simulink library "library_schuettgut"  (R2020a)
settings: Solver=VariableStepAuto  StartTime=0.0  StopTime=10.0  RelTol=1e-3
undefined symbols (not defined in the file or in its folder): alpha, beta, n_n, T, tau_LV, tau_OL, tau_SK, tau_V
libraries: simulink x9, powerlib_meascontrol x2
settings Model: Creator=Jonathan  LastModifiedBy=Jonathan

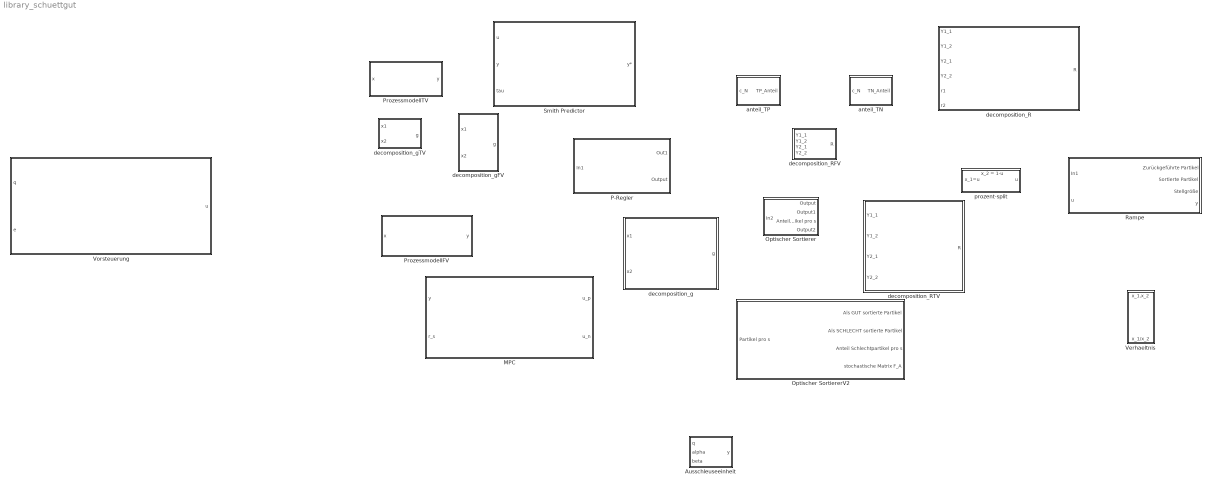
== system library_schuettgut ==
  Ausschleuseeinheit : MATLAB Function  TreatAsAtomicUnit=on
  MPC : Subsystem
  Optischer Sortierer : Subsystem  mask{alpha=0, beta=0}
      mask prompts: alpha "Wahrscheinlichkeit alpha:"; beta "Wahrscheinlichkeit beta:"
  Optischer SortiererV2 : Subsystem  AncestorBlock=library_schuettgut/Optischer Sortierer
  P-Regler : Subsystem  mask{gain=1, delay=1, TrueorFalse=0}
      mask prompts: delay "Time Delay"; TrueorFalse "Reglerinput"
  ProzessmodellFV : Subsystem
  ProzessmodellTV : Subsystem
  Rampe : Subsystem  Tag=Rampe  mask{OK=tau_OL, errorP=0, errorN=0, KV=tau_LV, V=tau_V, TrueorFalse=0, delay=0.2, gain=8.6, KP=6/10000, KN=6/10000}
      mask prompts: OK "Abstand OS Kamera"; errorP "Reglerfehler Gutpartikel:"; errorN "Reglerfehler Schlechtpartikel"; KV "Abstand Kamera Vakuumsauger"; V "Totzeit durch Absaugen"; TrueorFalse "Reglerinput:"; delay "Regler-Totzeit"; gain "Regler-Gain:"; KP "Amplitude des Kameramessrauschen für die positiven Partikel"; KN "Amplitude des Kameramessrauschen für die negativen Partikel"
      mask help:
      | Reglerinput:
      | Reglerinput = 1 => Gutpartikel pro s wird als Regelgröße verwendet
      | Reglerinput = 0 => Schlechtpartike pro s wird als Regelgröße verwendet
      mask TypeOptions TrueorFalse: 0 | 1
      mask DialogControl Regler Prompt: Regler
      mask DialogControl Kamera Prompt: Kamera
  Smith Predictor : Subsystem
  "Verhaeltnis " : Subsystem
  Vorsteuerung : Subsystem
  anteil_TN : MATLAB Function  TreatAsAtomicUnit=on
  anteil_TP : MATLAB Function  TreatAsAtomicUnit=on
  decomposition_R : MATLAB Function  TreatAsAtomicUnit=on
  decomposition_RFV : MATLAB Function  TreatAsAtomicUnit=on
  decomposition_RTV : MATLAB Function  TreatAsAtomicUnit=on
  decomposition_g : MATLAB Function  TreatAsAtomicUnit=on
  decomposition_gFV : MATLAB Function  TreatAsAtomicUnit=on
  decomposition_gTV : MATLAB Function  TreatAsAtomicUnit=on
  prozent-split : Subsystem
      settings: PortSchema="{\"entries\":[{\"content\":{\"sides\":[{\"content\":{\"connectorIds\":[\"In1\"]},\"type\":\"ConnectorPlacement.EquallySpacedRectSide\",\"uuid\":\"ab8511c8-9f1d-48ad-bf24-85fd477f0bdd\"},{\"content\":{\"connectorIds\":[\"Out1\"],\"side\":\"RIGHT\"},\"type\":\"ConnectorPlacement.EquallySpacedRectSide\",\"uuid\":\"9ac1a19a-8176-444e-9f4d-7beffa0184e3\"},{\"content\":{\"connectorIds\":[\"Out2\"],\"side\":\"TOP\"},\"type\":\"ConnectorPlacement.EquallySpacedRectSide\",\"uuid\":\"376c2400-f821-4649-ab16-706a2da6117b\"}]},\"type\":\"ConnectorPlacement.EquallySpacedConnector\",\"uuid\":\"f6e72b2d-0467-4732-a018-d51f3a5db703\"}],\"packageUris\":[\"http://schema.mathworks.com/mf0/Connector/19700101\"],\"version\":\"1.0\"}"

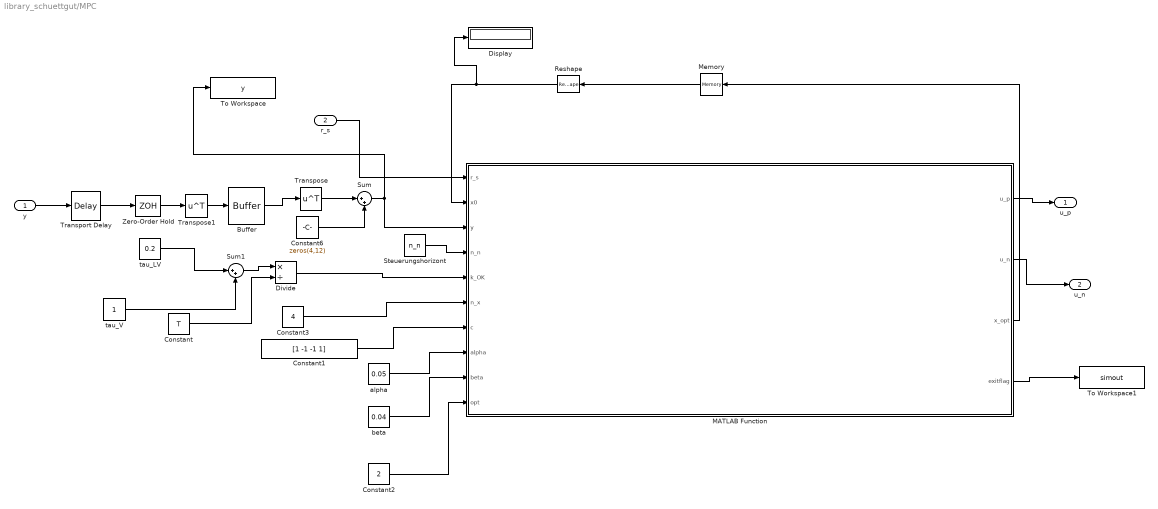
== system library_schuettgut/MPC ==
  y : Inport
  r_s : Inport  Port=2
  Buffer : Buffer  N=n_n  V=n_n-1  OutputFrames=off
  Constant : Constant  Value=T
  Constant1 : Constant  Value=[1 -1 -1 1]
  Constant2 : Constant  Value=2
  Constant3 : Constant  Value=4
  Constant6 : Constant  Value=zeros(4,12)
  Display : Display
  Divide : Product  Inputs=*/
  MATLAB Function : MATLAB Function  TreatAsAtomicUnit=on  SystemSampleTime=T
  Memory : Memory
  Reshape : Reshape  OutputDimensionality=Customize  OutputDimensions=[48,1]
  Steuerungshorizont : Constant  Value=n_n
  Sum : Sum  Inputs=|++
  Sum1 : Sum  Inputs=|++
  To Workspace : ToWorkspace  VariableName=y  SaveFormat=Timeseries  SampleTime=-1
  To Workspace1 : ToWorkspace  VariableName=simout  SaveFormat=Timeseries  SampleTime=-1
  Transport Delay : TransportDelay  DelayTime=tau_SK
  Transpose : Math  Operator=transpose  SaturateOnIntegerOverflow=on
  Transpose1 : Math  Operator=transpose  SaturateOnIntegerOverflow=on
  Zero-Order Hold : ZeroOrderHold  SampleTime=0.1
  alpha : Constant  Value=0.05
  beta : Constant  Value=0.04
  tau_LV : Constant  Value=0.2
  tau_V : Constant
  u_p : Outport
  u_n : Outport  Port=2
  wires:
  r_s/1 -> MATLAB Function/1(r_s)
  MATLAB Function/3(x_opt) -> Memory/1
  alpha/1 -> MATLAB Function/8(alpha)
  beta/1 -> MATLAB Function/9(beta)
  Constant1/1 -> MATLAB Function/7(c)
  Constant3/1 -> MATLAB Function/6(n_x)
  y/1 -> Transport Delay/1
  Zero-Order Hold/1 -> Transpose1/1
  Buffer/1 -> Transpose/1
  Constant6/1 -> Sum/2
  MATLAB Function/2(u_n) -> u_n/1
  MATLAB Function/1(u_p) -> u_p/1
  Transpose1/1 -> Buffer/1
  Memory/1 -> Reshape/1
  Reshape/1 -> MATLAB Function/2(x0), Display/1
  Sum/1 -> To Workspace/1, MATLAB Function/3(y)
  MATLAB Function/4(exitflag) -> To Workspace1/1
  Constant2/1 -> MATLAB Function/10(opt)
  tau_LV/1 -> Sum1/1
  tau_V/1 -> Sum1/2
  Sum1/1 -> Divide/1
  Divide/1 -> MATLAB Function/5(k_OK)
  Constant/1 -> Divide/2
  Transpose/1 -> Sum/1
  Steuerungshorizont/1 -> MATLAB Function/4(n_n)
  Transport Delay/1 -> Zero-Order Hold/1

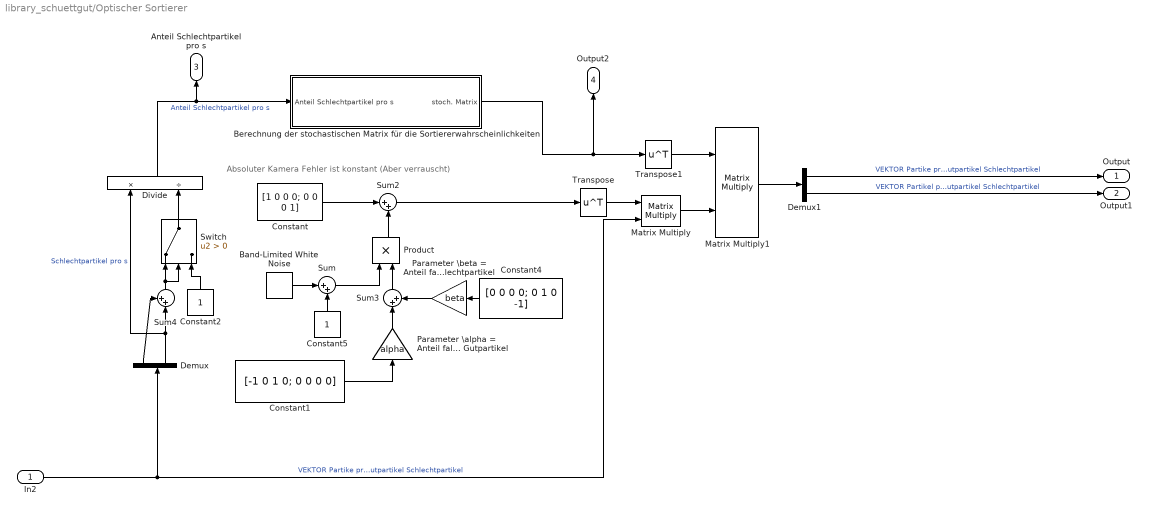
== system library_schuettgut/Optischer Sortierer ==
  note: Absoluter Kamera Fehler ist konstant (Aber verrauscht)
  In2 : Inport
  Band-Limited White Noise : simulink/Sources/Band-Limited White Noise  Cov=[0]  Ts=0.1  seed=[23341]
  Berechnung der stochastischen Matrix für die Sortiererwahrscheinlichkeiten : Subsystem
  Constant : Constant  Value=[1 0 0 0; 0 0 0 1]
  Constant1 : Constant  Value=[-1 0 1 0; 0 0 0 0]
  Constant2 : Constant
  Constant4 : Constant  Value=[0 0 0 0; 0 1 0 -1]
  Constant5 : Constant
  Demux : Demux  Outputs=2
  Demux1 : Demux  Outputs=2
  Divide : Product  Inputs=*/
  Matrix Multiply : Product  Multiplication=Matrix(*)
  Matrix Multiply1 : Product  Multiplication=Matrix(*)
  Parameter \alpha = Anteil falsch detektierter Gutpartikel : Gain  Gain=alpha
  Parameter \beta = Anteil falsch detektierter Schlechtpartikel : Gain  Gain=beta
  Product : Product
  Sum : Sum  Inputs=|++
  Sum2 : Sum  Inputs=|++
  Sum3 : Sum  Inputs=|++
  Sum4 : Sum  Inputs=++|
  Switch : Switch  Criteria=u2 > Threshold
  Transpose : Math  Operator=transpose  SaturateOnIntegerOverflow=on
  Transpose1 : Math  Operator=transpose  SaturateOnIntegerOverflow=on
  Output : Outport
  Output1 : Outport  Port=2
  Anteil Schlechtpartikel pro s : Outport  Port=3
  Output2 : Outport  Port=4
  wires:
  Constant2/1 -> Switch/3
  Switch/1 -> Divide/2
  Constant5/1 -> Sum/2
  Band-Limited White Noise/1 -> Sum/1
  Sum/1 -> Product/1
  Product/1 -> Sum2/2
  Constant/1 -> Sum2/1
  Sum3/1 -> Product/2
  Parameter \alpha = Anteil falsch detektierter Gutpartikel/1 -> Sum3/1
  Parameter \beta = Anteil falsch detektierter Schlechtpartikel/1 -> Sum3/2
  Constant4/1 -> Parameter \beta = Anteil falsch detektierter Schlechtpartikel/1
  Berechnung der stochastischen Matrix für die Sortiererwahrscheinlichkeiten/1(stoch. Matrix) -> Transpose1/1, Output2/1
  Divide/1 -> Berechnung der stochastischen Matrix für die Sortiererwahrscheinlichkeiten/1(Anteil Schlechtpartikel pro s), Anteil Schlechtpartikel pro s/1  "Anteil Schlechtpartikel pro s"
  Demux/1 -> Sum4/1
  Sum4/1 -> Switch/1, Switch/2
  Demux/2 -> Sum4/2, Divide/1  "Schlechtpartikel pro s"
  Sum2/1 -> Transpose/1
  Constant1/1 -> Parameter \alpha = Anteil falsch detektierter Gutpartikel/1
  In2/1 -> Demux/1, Matrix Multiply/2  "VEKTOR Partike pro s: Gutpartikel Schlechtpartikel"
  Matrix Multiply1/1 -> Demux1/1
  Transpose1/1 -> Matrix Multiply1/1
  Matrix Multiply/1 -> Matrix Multiply1/2
  Transpose/1 -> Matrix Multiply/1
  Demux1/2 -> Output1/1  "VEKTOR Partikel pro s in der Schlechtfraktion: Gutpartikel Schlechtpartikel"
  Demux1/1 -> Output/1  "VEKTOR Partike pro s in der Gutfraktion: Gutpartikel Schlechtpartikel"

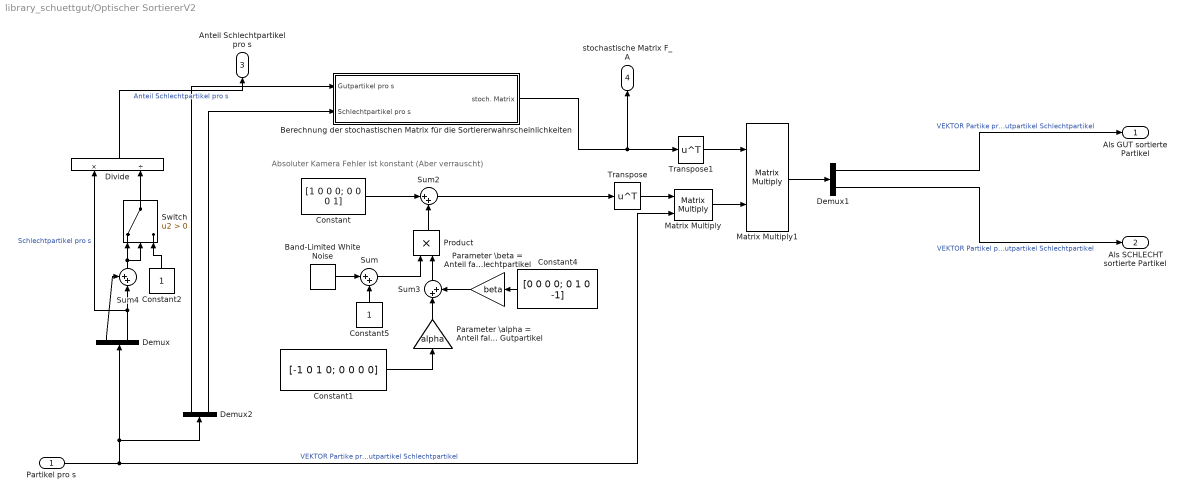
== system library_schuettgut/Optischer SortiererV2 ==
  note: Absoluter Kamera Fehler ist konstant (Aber verrauscht)
  Partikel pro s : Inport
  Band-Limited White Noise : simulink/Sources/Band-Limited White Noise  Cov=[0]  Ts=0.1  seed=[23341]
  Berechnung der stochastischen Matrix für die Sortiererwahrscheinlichkeiten : Subsystem
  Constant : Constant  Value=[1 0 0 0; 0 0 0 1]
  Constant1 : Constant  Value=[-1 0 1 0; 0 0 0 0]
  Constant2 : Constant
  Constant4 : Constant  Value=[0 0 0 0; 0 1 0 -1]
  Constant5 : Constant
  Demux : Demux  Outputs=2
  Demux1 : Demux  Outputs=2
  Demux2 : Demux  Outputs=2
  Divide : Product  Inputs=*/
  Matrix Multiply : Product  Multiplication=Matrix(*)
  Matrix Multiply1 : Product  Multiplication=Matrix(*)
  Parameter \alpha = Anteil falsch detektierter Gutpartikel : Gain  Gain=alpha
  Parameter \beta = Anteil falsch detektierter Schlechtpartikel : Gain  Gain=beta
  Product : Product
  Sum : Sum  Inputs=|++
  Sum2 : Sum  Inputs=|++
  Sum3 : Sum  Inputs=|++
  Sum4 : Sum  Inputs=++|
  Switch : Switch  Criteria=u2 > Threshold
  Transpose : Math  Operator=transpose  SaturateOnIntegerOverflow=on
  Transpose1 : Math  Operator=transpose  SaturateOnIntegerOverflow=on
  Als GUT sortierte Partikel : Outport
  Als SCHLECHT sortierte Partikel : Outport  Port=2
  Anteil Schlechtpartikel pro s : Outport  Port=3
  stochastische Matrix F_A : Outport  Port=4
  wires:
  Demux1/1 -> Als GUT sortierte Partikel/1  "VEKTOR Partike pro s in der Gutfraktion: Gutpartikel Schlechtpartikel"
  Demux1/2 -> Als SCHLECHT sortierte Partikel/1  "VEKTOR Partikel pro s in der Schlechtfraktion: Gutpartikel Schlechtpartikel"
  Transpose/1 -> Matrix Multiply/1
  Matrix Multiply/1 -> Matrix Multiply1/2
  Transpose1/1 -> Matrix Multiply1/1
  Matrix Multiply1/1 -> Demux1/1
  Partikel pro s/1 -> Matrix Multiply/2, Demux2/1, Demux/1  "VEKTOR Partike pro s: Gutpartikel Schlechtpartikel"
  Constant1/1 -> Parameter \alpha = Anteil falsch detektierter Gutpartikel/1
  Sum2/1 -> Transpose/1
  Demux/2 -> Divide/1, Sum4/2  "Schlechtpartikel pro s"
  Sum4/1 -> Switch/2, Switch/1
  Demux/1 -> Sum4/1
  Divide/1 -> Anteil Schlechtpartikel pro s/1  "Anteil Schlechtpartikel pro s"
  Berechnung der stochastischen Matrix für die Sortiererwahrscheinlichkeiten/1(stoch. Matrix) -> stochastische Matrix F_A/1, Transpose1/1
  Constant4/1 -> Parameter \beta = Anteil falsch detektierter Schlechtpartikel/1
  Parameter \beta = Anteil falsch detektierter Schlechtpartikel/1 -> Sum3/2
  Parameter \alpha = Anteil falsch detektierter Gutpartikel/1 -> Sum3/1
  Sum3/1 -> Product/2
  Constant/1 -> Sum2/1
  Product/1 -> Sum2/2
  Sum/1 -> Product/1
  Band-Limited White Noise/1 -> Sum/1
  Constant5/1 -> Sum/2
  Switch/1 -> Divide/2
  Constant2/1 -> Switch/3
  Demux2/1 -> Berechnung der stochastischen Matrix für die Sortiererwahrscheinlichkeiten/1(Gutpartikel pro s)
  Demux2/2 -> Berechnung der stochastischen Matrix für die Sortiererwahrscheinlichkeiten/2(Schlechtpartikel pro s)

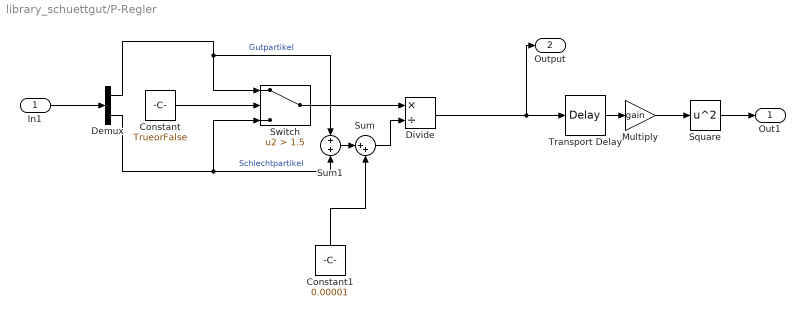
== system library_schuettgut/P-Regler ==
  In1 : Inport
  Constant : Constant  Value=TrueorFalse
  Constant1 : Constant  Value=0.00001
  Demux : Demux  Outputs=2
  Divide : Product  Inputs=*/
  Multiply : Gain  Gain=gain
  Square : Math  Operator=square  SaturateOnIntegerOverflow=on
  Sum : Sum  Inputs=|++
  Sum1 : Sum  Inputs=+|+
  Switch : Switch  Criteria=u2 > Threshold  Threshold=1.5
  Transport Delay : TransportDelay  DelayTime=delay
  Out1 : Outport
  Output : Outport  Port=2
  wires:
  In1/1 -> Demux/1
  Demux/2 -> Switch/3, Sum1/2  "Schlechtpartikel"
  Transport Delay/1 -> Multiply/1
  Multiply/1 -> Square/1
  Constant/1 -> Switch/2
  Demux/1 -> Sum1/1, Switch/1  "Gutpartikel"
  Sum1/1 -> Sum/1
  Sum/1 -> Divide/2
  Constant1/1 -> Sum/2
  Switch/1 -> Divide/1
  Divide/1 -> Transport Delay/1, Output/1
  Square/1 -> Out1/1

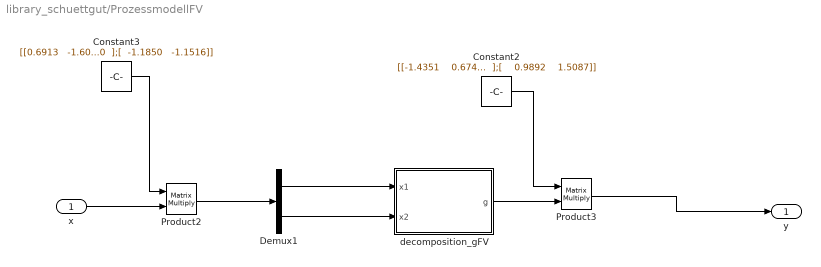
== system library_schuettgut/ProzessmodellFV ==
  x : Inport
  Constant2 : Constant  Value=|
      | [[-1.4351    0.6740
      |  ];[    0.9892    1.5087]]
  Constant3 : Constant  Value=|
      | [[0.6913   -1.6000
      |  ];[  -1.1850   -1.1516]]
  Demux1 : Demux  Outputs=2
  Product2 : Product  Multiplication=Matrix(*)
  Product3 : Product  Multiplication=Matrix(*)
  decomposition_gFV : MATLAB Function  TreatAsAtomicUnit=on
  y : Outport
  wires:
  Constant3/1 -> Product2/1
  Product2/1 -> Demux1/1
  Product3/1 -> y/1
  Constant2/1 -> Product3/1
  Demux1/2 -> decomposition_gFV/2(x2)
  Demux1/1 -> decomposition_gFV/1(x1)
  decomposition_gFV/1(g) -> Product3/2
  x/1 -> Product2/2

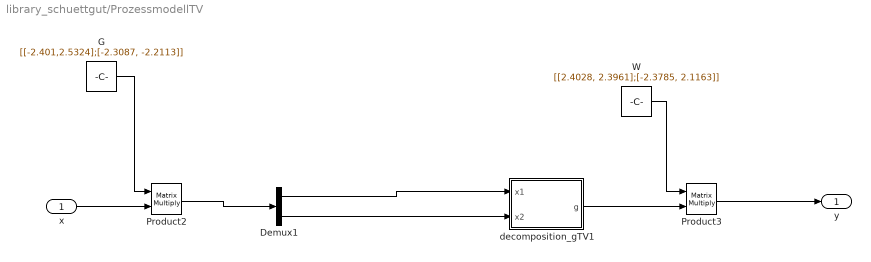
== system library_schuettgut/ProzessmodellTV ==
  x : Inport
  Demux1 : Demux  Outputs=2
  G : Constant  Value=[[-2.401,2.5324];[-2.3087, -2.2113]]
  Product2 : Product  Multiplication=Matrix(*)
  Product3 : Product  Multiplication=Matrix(*)
  W : Constant  Value=[[2.4028, 2.3961];[-2.3785, 2.1163]]
  decomposition_gTV1 : MATLAB Function  TreatAsAtomicUnit=on
  y : Outport
  wires:
  G/1 -> Product2/1
  Demux1/1 -> decomposition_gTV1/1(x1)
  Product3/1 -> y/1
  Product2/1 -> Demux1/1
  x/1 -> Product2/2
  Demux1/2 -> decomposition_gTV1/2(x2)
  W/1 -> Product3/1
  decomposition_gTV1/1(g) -> Product3/2

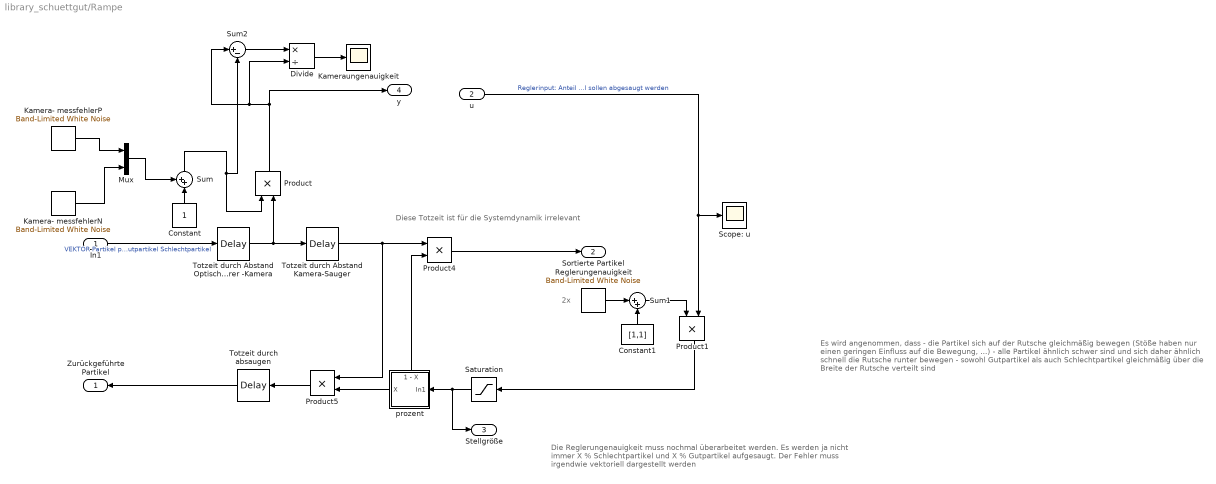
== system library_schuettgut/Rampe ==
  note: Diese Totzeit ist für die Systemdynamik irrelevant
  note: 2x
  note: Die Reglerungenauigkeit muss nochmal überarbeitet werden.
      | Es werden ja nicht immer X % Schlechtpartikel und X %
      | Gutpartikel aufgesaugt. Der Fehler muss irgendwie vektoriell dargestellt werden
  note: Es wird angenommen, dass
      | - die Partikel sich auf der Rutsche gleichmäßig bewegen (Stöße haben nur einen geringen Einfluss auf die Bewegung, ...)
      | - alle Partikel ähnlich schwer sind und sich daher ähnlich schnell die Rutsche runter bewegen
      | - sowohl Gutpartikel als auch Schlechtpartikel gleichmäßig über die Breite der Rutsche verteilt sind
  In1 : Inport
  u : Inport  Port=2
  Constant : Constant
  Constant1 : Constant  Value=[1,1]
  Divide : Product  Inputs=*/
  Kamera- messfehlerN : simulink/Sources/Band-Limited White Noise  Cov=[KN]  Ts=0.6  seed=[242211]
  Kamera- messfehlerP : simulink/Sources/Band-Limited White Noise  Cov=[KP]  Ts=0.6  seed=[15432]
  Kameraungenauigkeit : Scope
  Mux : Mux  Inputs=2
  Product : Product
  Product1 : Product  OutMin=0  OutMax=1
  Product4 : Product
  Product5 : Product
  Reglerungenauigkeit : simulink/Sources/Band-Limited White Noise  Cov=[errorP errorN]  Ts=0.1  seed=[23341]
  Saturation : Saturate  UpperLimit=1  LowerLimit=0
  Scope: u : Scope
  Sum : Sum  Inputs=++|
  Sum1 : Sum  Inputs=|++
  Sum2 : Sum  Inputs=|+-
  Totzeit durch Abstand Optischer Sortierer -Kamera : TransportDelay  DelayTime=OK
  Totzeit durch Abstand Kamera-Sauger : TransportDelay  DelayTime=KV
  Totzeit durch absaugen : TransportDelay  DelayTime=V
  prozent : Subsystem
      settings: PortSchema="{\"entries\":[{\"content\":{\"sides\":[{\"content\":{\"connectorIds\":[\"In1\"]},\"type\":\"ConnectorPlacement.EquallySpacedRectSide\",\"uuid\":\"ab8511c8-9f1d-48ad-bf24-85fd477f0bdd\"},{\"content\":{\"connectorIds\":[\"Out1\"],\"side\":\"RIGHT\"},\"type\":\"ConnectorPlacement.EquallySpacedRectSide\",\"uuid\":\"9ac1a19a-8176-444e-9f4d-7beffa0184e3\"},{\"content\":{\"connectorIds\":[\"Out2\"],\"side\":\"TOP\"},\"type\":\"ConnectorPlacement.EquallySpacedRectSide\",\"uuid\":\"376c2400-f821-4649-ab16-706a2da6117b\"}]},\"type\":\"ConnectorPlacement.EquallySpacedConnector\",\"uuid\":\"f6e72b2d-0467-4732-a018-d51f3a5db703\"}],\"packageUris\":[\"http://schema.mathworks.com/mf0/Connector/19700101\"],\"version\":\"1.0\"}"
  Zurückgeführte Partikel : Outport
  Sortierte Partikel : Outport  Port=2
  Stellgröße : Outport  Port=3
  y : Outport  Port=4
  wires:
  prozent/2(1 - X) -> Product4/2
  prozent/1(X) -> Product5/2
  In1/1 -> Totzeit durch Abstand Optischer Sortierer -Kamera/1  "VEKTOR Partikel pro s: Gutpartikel Schlechtpartikel"
  Product/1 -> Divide/2, Sum2/1, y/1
  Totzeit durch absaugen/1 -> Zurückgeführte Partikel/1
  Totzeit durch Abstand Optischer Sortierer -Kamera/1 -> Totzeit durch Abstand Kamera-Sauger/1, Product/2
  Product5/1 -> Totzeit durch absaugen/1
  Product4/1 -> Sortierte Partikel/1
  Kamera- messfehlerN/1 -> Mux/2
  u/1 -> Scope: u/1, Product1/2  "Reglerinput: Anteil X der Partikel sollen abgesaugt werden"
  Constant/1 -> Sum/2
  Sum/1 -> Sum2/2, Product/1
  Reglerungenauigkeit/1 -> Sum1/1
  Constant1/1 -> Sum1/2
  Product1/1 -> Saturation/1
  Saturation/1 -> Stellgröße/1, prozent/1(In1)
  Sum1/1 -> Product1/1
  Totzeit durch Abstand Kamera-Sauger/1 -> Product4/1, Product5/1
  Kamera- messfehlerP/1 -> Mux/1
  Mux/1 -> Sum/1
  Sum2/1 -> Divide/1
  Divide/1 -> Kameraungenauigkeit/1

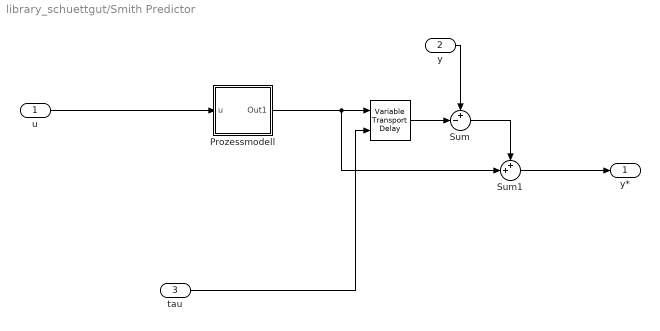
== system library_schuettgut/Smith Predictor ==
  u : Inport
  y : Inport  Port=2
  tau : Inport  Port=3
  " " : VariableTransportDelay  VariableDelayType=Variable transport delay  MaximumDelay=10  MaximumPoints=30000
  Prozessmodell : Subsystem
  Sum : Sum  Inputs=+-|
  Sum1 : Sum  Inputs=++|
  y* : Outport
  wires:
  Prozessmodell/1(Out1) -> Sum1/2, " "/1
  " "/1 -> Sum/2
  y/1 -> Sum/1
  Sum1/1 -> y*/1
  Sum/1 -> Sum1/1
  tau/1 -> " "/2
  u/1 -> Prozessmodell/1(u)

== system library_schuettgut/Verhaeltnis  ==
  x_1,x_2 : Inport
  Demux : Demux  Outputs=2
  Divide : Product  Inputs=*/
  Sum : Sum  Inputs=++|
  x_1/x_2 : Outport
  wires:
  Divide/1 -> x_1/x_2/1
  Demux/2 -> Sum/2
  Demux/1 -> Divide/1, Sum/1
  x_1,x_2/1 -> Demux/1
  Sum/1 -> Divide/2

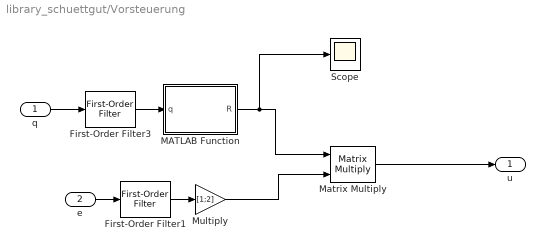
== system library_schuettgut/Vorsteuerung ==
  q : Inport
  e : Inport  Port=2
  First-Order Filter1 : powerlib_meascontrol/Filters/First-Order Filter  FilterType=Lowpass  Tc=200  Ts=0  Initialize=off  Vac_Init=[0, 0, 60]  Vdc_Init=0  PlotResponse=off  FreqRange="[0,  200,  1]"
  First-Order Filter3 : powerlib_meascontrol/Filters/First-Order Filter  FilterType=Lowpass  Tc=200  Ts=0  Initialize=off  Vac_Init=[0, 0, 60]  Vdc_Init=0  PlotResponse=off  FreqRange="[0,  200,  1]"
  MATLAB Function : MATLAB Function  TreatAsAtomicUnit=on
  Matrix Multiply : Product  Multiplication=Matrix(*)
  Multiply : Gain  Gain=[1;2]
  Scope : Scope
  u : Outport
  wires:
  MATLAB Function/1(R) -> Scope/1, Matrix Multiply/1
  q/1 -> First-Order Filter3/1
  Matrix Multiply/1 -> u/1
  e/1 -> First-Order Filter1/1
  Multiply/1 -> Matrix Multiply/2
  First-Order Filter3/1 -> MATLAB Function/1(q)
  First-Order Filter1/1 -> Multiply/1

== system library_schuettgut/prozent-split ==
  u : Inport
  Constant3 : Constant
  Sum7 : Sum  Inputs=|-+
  x_1=u : Outport
  x_2 = 1-u : Outport  Port=2
  wires:
  Constant3/1 -> Sum7/2
  u/1 -> Sum7/1, x_1=u/1  "Reglerinput"
  Sum7/1 -> x_2 = 1-u/1

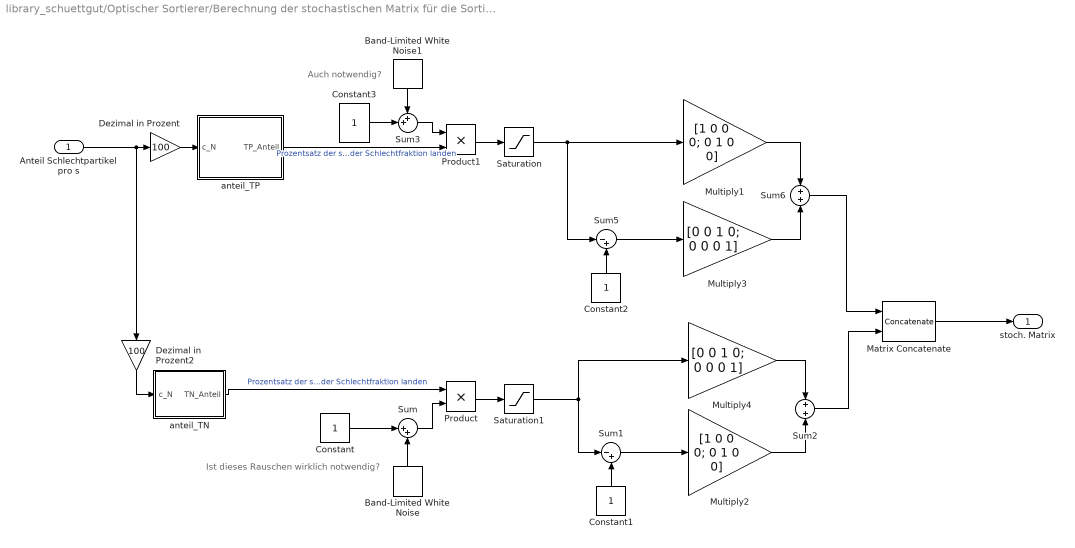
== system library_schuettgut/Optischer Sortierer/Berechnung der stochastischen Matrix für die Sortiererwahrscheinlichkeiten ==
  note: Ist dieses Rauschen wirklich notwendig?
  note: Auch notwendig?
  Anteil Schlechtpartikel pro s : Inport
  Band-Limited White Noise : simulink/Sources/Band-Limited White Noise  Cov=[0]  Ts=0.1  seed=[23341]
  Band-Limited White Noise1 : simulink/Sources/Band-Limited White Noise  Cov=[0]  Ts=0.1  seed=[23341]
  Constant{,1..3} (4 alike) : Constant
  Dezimal in Prozent : Gain  Gain=100
  Dezimal in Prozent2 : Gain  Gain=100
  Matrix Concatenate : Concatenate  Mode=Multidimensional array
  Multiply1 : Gain  Gain=[1 0 0 0; 0 1 0 0]
  Multiply2 : Gain  Gain=[1 0 0 0; 0 1 0 0]
  Multiply3 : Gain  Gain=[0 0 1 0; 0 0 0 1]
  Multiply4 : Gain  Gain=[0 0 1 0; 0 0 0 1]
  Product : Product
  Product1 : Product
  Saturation : Saturate  UpperLimit=1  LowerLimit=0
  Saturation1 : Saturate  UpperLimit=1  LowerLimit=0
  Sum : Sum  Inputs=|++
  Sum1 : Sum  Inputs=|-+
  Sum2 : Sum  Inputs=+|+
  Sum3 : Sum  Inputs=++|
  Sum5 : Sum  Inputs=|-+
  Sum6 : Sum  Inputs=+|+
  anteil_TN : MATLAB Function  TreatAsAtomicUnit=on
  anteil_TP : MATLAB Function  TreatAsAtomicUnit=on
  stoch. Matrix : Outport
  wires:
  Band-Limited White Noise/1 -> Sum/2
  Product/1 -> Saturation1/1
  Product1/1 -> Saturation/1
  Band-Limited White Noise1/1 -> Sum3/1
  anteil_TP/1(TP_Anteil) -> Product1/2  "Prozentsatz der schlecht detektierten Partikel, die in der Schlechtfraktion landen"
  anteil_TN/1(TN_Anteil) -> Product/1  "Prozentsatz der schlecht detektierten Partikel, die in der Schlechtfraktion landen"
  Constant3/1 -> Sum3/2
  Sum3/1 -> Product1/1
  Constant/1 -> Sum/1
  Sum/1 -> Product/2
  Dezimal in Prozent2/1 -> anteil_TN/1(c_N)
  Dezimal in Prozent/1 -> anteil_TP/1(c_N)
  Saturation/1 -> Multiply1/1, Sum5/1
  Saturation1/1 -> Sum1/1, Multiply4/1
  Sum6/1 -> Matrix Concatenate/1
  Sum2/1 -> Matrix Concatenate/2
  Matrix Concatenate/1 -> stoch. Matrix/1
  Multiply1/1 -> Sum6/1
  Anteil Schlechtpartikel pro s/1 -> Dezimal in Prozent2/1, Dezimal in Prozent/1
  Multiply4/1 -> Sum2/1
  Multiply2/1 -> Sum2/2
  Constant1/1 -> Sum1/2
  Sum1/1 -> Multiply2/1
  Constant2/1 -> Sum5/2
  Sum5/1 -> Multiply3/1
  Multiply3/1 -> Sum6/2

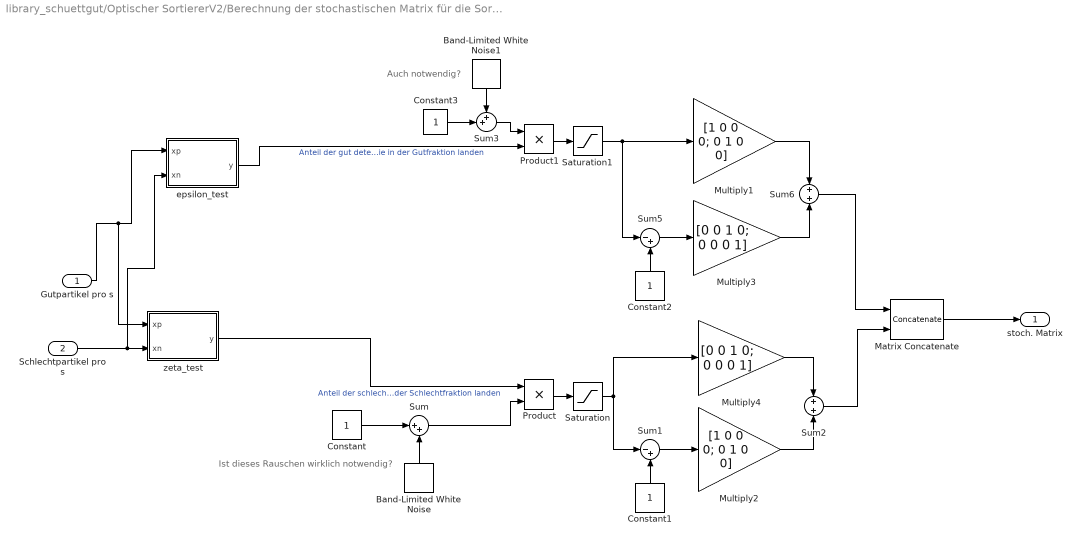
== system library_schuettgut/Optischer SortiererV2/Berechnung der stochastischen Matrix für die Sortiererwahrscheinlichkeiten ==
  note: Auch notwendig?
  note: Ist dieses Rauschen wirklich notwendig?
  Gutpartikel pro s : Inport
  Schlechtpartikel pro s : Inport  Port=2
  Band-Limited White Noise : simulink/Sources/Band-Limited White Noise  Cov=[0]  Ts=0.1  seed=[23341]
  Band-Limited White Noise1 : simulink/Sources/Band-Limited White Noise  Cov=[0]  Ts=0.1  seed=[23341]
  Constant{,1..3} (4 alike) : Constant
  Matrix Concatenate : Concatenate  Mode=Multidimensional array
  Multiply1 : Gain  Gain=[1 0 0 0; 0 1 0 0]
  Multiply2 : Gain  Gain=[1 0 0 0; 0 1 0 0]
  Multiply3 : Gain  Gain=[0 0 1 0; 0 0 0 1]
  Multiply4 : Gain  Gain=[0 0 1 0; 0 0 0 1]
  Product : Product
  Product1 : Product
  Saturation : Saturate  UpperLimit=1  LowerLimit=0
  Saturation1 : Saturate  UpperLimit=1  LowerLimit=0
  Sum : Sum  Inputs=|++
  Sum1 : Sum  Inputs=|-+
  Sum2 : Sum  Inputs=+|+
  Sum3 : Sum  Inputs=++|
  Sum5 : Sum  Inputs=|-+
  Sum6 : Sum  Inputs=+|+
  epsilon_test : MATLAB Function  TreatAsAtomicUnit=on
  zeta_test : MATLAB Function  TreatAsAtomicUnit=on
  stoch. Matrix : Outport
  wires:
  Multiply3/1 -> Sum6/2
  Sum5/1 -> Multiply3/1
  Constant2/1 -> Sum5/2
  Sum1/1 -> Multiply2/1
  Constant1/1 -> Sum1/2
  Multiply2/1 -> Sum2/2
  Multiply4/1 -> Sum2/1
  Multiply1/1 -> Sum6/1
  Matrix Concatenate/1 -> stoch. Matrix/1
  Sum2/1 -> Matrix Concatenate/2
  Sum6/1 -> Matrix Concatenate/1
  Product/1 -> Saturation/1
  Product1/1 -> Saturation1/1
  Sum/1 -> Product/2
  Constant/1 -> Sum/1
  Sum3/1 -> Product1/1
  Constant3/1 -> Sum3/2
  zeta_test/1(y) -> Product/1  "Anteil der schlecht detektierten Partikel, die in der Schlechtfraktion landen"
  epsilon_test/1(y) -> Product1/2  "Anteil der gut detektierten Partikel, die in der Gutfraktion landen"
  Band-Limited White Noise1/1 -> Sum3/1
  Band-Limited White Noise/1 -> Sum/2
  Gutpartikel pro s/1 -> zeta_test/1(xp), epsilon_test/1(xp)
  Schlechtpartikel pro s/1 -> zeta_test/2(xn), epsilon_test/2(xn)
  Saturation/1 -> Multiply4/1, Sum1/1
  Saturation1/1 -> Sum5/1, Multiply1/1

== system library_schuettgut/Rampe/prozent ==
  In1 : Inport
  Constant3 : Constant
  Sum7 : Sum  Inputs=|-+
  X : Outport
  1 - X : Outport  Port=2
  wires:
  Constant3/1 -> Sum7/2
  In1/1 -> Sum7/1, X/1  "Reglerinput"
  Sum7/1 -> 1 - X/1

== system library_schuettgut/Smith Predictor/Prozessmodell ==
  u : Inport
  Out1 : Outport
  wires:
  u/1 -> Out1/1

== matlab function library_schuettgut/decomposition_g ==
  data: x1 input; g output; x2 input
function g = decomposition_g(x1,x2)
%#codegen

%    This function was generated by the Symbolic Math Toolbox version 8.5.
%    23-Jan-2021 16:21:08

t2 = conj(x1);
t3 = conj(x2);
g = [t2.*7.356750433682986e-2-t2.^2.*1.321341967872517e-2+7.302013683153394e-1;t3.*(-6.207010509479585e-2)-t3.^2.*6.60820597936792e-3+8.465045474029088e-1];

== matlab function library_schuettgut/decomposition_R ==
  data: Y1_1 input; R output; Y1_2 input; Y2_1 input; Y2_2 input; r1 input; r2 input
function R = decomposition_R(Y1_1,Y1_2,Y2_1,Y2_2,r1,r2)
%#codegen

%    This function was generated by the Symbolic Math Toolbox version 8.5.
%    23-Jan-2021 16:21:20

t2 = Y1_1.*Y2_2;
t3 = Y1_2.*Y2_1;
t4 = -t3;
t5 = t2+t4;
t6 = 1.0./t5;
R = reshape([r1.*(Y1_1.*t6.*4.209654314594556e-1-Y1_2.*t6.*2.514923794238454e-1-Y2_1.*t6.*2.36103808622674e-1+Y2_2.*t6.*1.41052695029348e-1), ...
r1.*(Y1_1.*t6.*1.329681620461174e-1-Y1_2.*t6.*5.885251943491074e-1-Y2_1.*t6.*7.457688241954584e-2+Y2_2.*t6.*3.300818296991368e-1),...
-r2.*(Y1_1.*t6.*9.471435133466113e-2-Y1_2.*t6.*5.658407033603224e-2-Y2_1.*t6.*5.862694938528591e-1+Y2_2.*t6.*3.502480226974876e-1),...
-r2.*(Y1_1.*t6.*2.991692969348502e-2-Y1_2.*t6.*1.324141553229882e-1-Y2_1.*t6.*1.851818967440092e-1+Y2_2.*t6.*8.196263684039293e-1)],[2,2]);
R(isnan(R))=0;
R(isinf(R))=100;

== matlab function library_schuettgut/decomposition_RTV ==
  data: Y1_1 input; R output; Y1_2 input; Y2_1 input; Y2_2 input
function R = decomposition_RTV(Y1_1,Y1_2,Y2_1,Y2_2)
%#codegen

%    This function was generated by the Symbolic Math Toolbox version 8.5.
%    26-Jan-2021 10:32:41

R = reshape([Y1_2.*(-2.137674923372295e-1)-Y2_2.*2.047522987447861e-1,Y1_1.*2.137674923372295e-1+Y2_1.*2.047522987447861e-1,Y1_2.*2.074157501900618e-1-Y2_2.*2.344807267266782e-1,Y1_1.*(-2.074157501900618e-1)+Y2_1.*2.344807267266782e-1],[2,2]);

== matlab function library_schuettgut/Vorsteuerung/MATLAB Function ==
  data: q input; R output
function R = fcn(q)
% q ist ein 4x1 Vektor mit q_TP,q_FP,q_FN,q_TN
Q_det = 1/(q(1)*q(4)-q(2)*q(3));
R = Q_det*[[q(4) -q(3)];[-q(2) q(1)]];
R(isnan(R)) = 0;
R(isinf(R)) = 10;

== matlab function library_schuettgut/decomposition_RFV ==
  data: Y1_1 input; R output; Y1_2 input; Y2_1 input; Y2_2 input
function R = decomposition_RFV(Y1_1,Y1_2,Y2_1,Y2_2)
%#codegen

%    This function was generated by the Symbolic Math Toolbox version 8.5.
%    27-Jan-2021 00:16:44

t2 = Y1_1.*Y2_2;
t3 = Y1_2.*Y2_1;
t4 = -t3;
t5 = t2+t4;
t6 = 1.0./t5;
R = reshape([(t6.*(Y1_2.*1.242776054276755e+15+Y2_2.*2.008792984723099e+15))./1.7592186044416e+13,t6.*(Y1_1.*1.242776054276755e+15+Y2_1.*2.008792984723099e+15).*(-5.684341886080801e-14),t6.*(Y1_2.*4.4187595480969e+13+Y2_2.*1.754353506433e+13).*(-1.63424829224823e-12),t6.*(Y1_1.*4.4187595480969e+13+Y2_1.*1.754353506433e+13).*1.63424829224823e-12],[2,2]);
R(isnan(R)) = 0;
R(isinf(R)) = 10;

== matlab function library_schuettgut/decomposition_gFV ==
  data: x1 input; g output; x2 input
function g = decomposition_gFV(x1,x2)
%#codegen

%    This function was generated by the Symbolic Math Toolbox version 8.5.
%    26-Jan-2021 22:17:03

g = [conj(x1).*(-1.377937986499028e-2)+1.601570395857327e-1;conj(x2).*1.81125395555236e-2+8.513571412265965e-2];

== matlab function library_schuettgut/ProzessmodellTV/decomposition_gTV1 ==
  data: x1 input; g output; x2 input
function g = decomposition_gTV(x1,x2)
%#codegen

%    This function was generated by the Symbolic Math Toolbox version 8.5.
%    26-Jan-2021 10:32:40

t2 = conj(x1);
t3 = conj(x2);
g = [t2.*(-6.586048041173689e-2)+t2.^2.*7.024962657286325e-5;t3.*(-1.448698496758973e-1)-t3.^2.*4.647981435157282e-3];

== matlab function library_schuettgut/Ausschleuseeinheit ==
  data: q input; y output; alpha input; beta input
function y = fcn(q,alpha, beta)
% Partikel auf dem Fließband
p = q(1); 
n = q(2);
% epsilon
p1 =   -0.003787;
p2 =     0.05479;
p3 =      0.6837;
p4 = -0.007;
epsilon = p1*(p+n).^2 + p2*(p+n) + p3 +p4*n;
% zeta
o1 =   -0.003787;
o2 =     0.05479;
o3 =      0.5837;
o4 = 0.007;
zeta = o1*(p+n).^2 + o2*(p+n) + o3 +o4*n;
% Partikel auf der Rutsche
fp = (beta*epsilon+(1-beta)*(1-zeta)).*n;
fn = (alpha*zeta+(1-alpha)*(1-epsilon)).*p;
tp = p - fn;
tn = n - fp;
y = [tp; fp; fn; tn];

== matlab function library_schuettgut/anteil_TN ==
  data: c_N input; TN_Anteil output
function TN_Anteil = anteil_TN(c_N)
%#codegen

%    This function was generated by the Symbolic Math Toolbox version 8.5.
%    10-Dec-2020 18:32:05

t2 = c_N.^2;
t3 = c_N.*1.216153139981487e-1;
t5 = c_N.*1.71830598234818e-4;
t4 = exp(t3);
t6 = -t5;
t7 = exp(t6);
TN_Anteil = ((c_N.*7.031194281766733e+17-t2.*8.263716299513051e+15+2.37569253023828e+20).*(c_N.*1.475739525896764e+20-t4.*1.784484509055505e+17+t7.*1.327876196767409e+22-1.475739525896764e+22).*(-1.355252715606881e-20))./(c_N.*(c_N.*-1.406238856353347e+18+t2.*1.65274325990261e+16+t4.*7.137938036222019e+15-t7.*5.311504787069636e+20+1.151573043110496e+20));

== matlab function library_schuettgut/anteil_TP ==
  data: c_N input; TP_Anteil output
function TP_Anteil = anteil_TP(c_N)
%#codegen

%    This function was generated by the Symbolic Math Toolbox version 8.5.
%    10-Dec-2020 18:32:05

t2 = c_N.^2;
t3 = c_N.*1.216153139981487e-1;
t5 = c_N.*1.71830598234818e-4;
t4 = exp(t3);
t6 = -t5;
t7 = exp(t6);
t8 = t4.*7.137938036222019e+15;
t9 = t7.*5.311504787069636e+20;
t10 = -t9;
TP_Anteil = ((t8+t10).*(c_N.*5.620899059042137e+19+t2.*2.065929074878263e+17-5.939231325595701e+21).*9.825582188149884e-19)./((c_N.*(1.45e+2./2.0)-7.25e+3).*(c_N.*-1.406238856353347e+18+t2.*1.65274325990261e+16+t8+t10+1.151573043110496e+20));

== matlab function library_schuettgut/ProzessmodellFV/decomposition_gFV ==
  data: x1 input; g output; x2 input
function g = decomposition_gFV(x1,x2)
%#codegen

%    This function was generated by the Symbolic Math Toolbox version 8.5.
%    26-Jan-2021 14:55:33

g = [conj(x1).*7.313115830678771e-2;conj(x2).*(-6.736451993880752e-2)];

== matlab function library_schuettgut/MPC/MATLAB Function ==
  data: u_p output; u_n output; r_s input; x_opt output; x0 input; y input; n_n input; k_OK input; n_x input; c input; alpha input; beta input; exitflag output; opt input
function [u_p,u_n, x_opt,exitflag]  = mpc(r_s, x0, y, n_n, k_OK, n_x, c, alpha, beta, opt)
%MPC Modellprädiktiver Regler für die Regelung einer Partikelrückführung
%für einen optischen Schüttgutsortierer.
%   Input:
%      -r_s: Matrix mit den Dimensionen 2,P; 
%       Dabei handelt es sich um die Vorhersage wie viele Gutpartikel 
%       (1. Zeile) und wie viele Schlechtpartikel (2. Zeile) von 
%       vorhergegangenen Prozessen auf das Fließband fallen
%      -x0: Optimale Steuergrößenfolge aus der letzten Optimierung, die
%       als Startwert für die kommende Optimierung genutzt wird.
%      -r_linie_old: Matrix mit den Dimensionen 4,1:
%       Anzahl Partikel die pro s zu den letzten k_OV Zeitpunkten auf der 
%       Rutsche fließen aufgeteilt nach:
%           -1. Zeile: Gutpartikel auf der Gutpartikelrutsche (TP)
%           -2. Zeile: Schlechtpartikel auf der Gutpartikelrutsche (FP)
%           -3. Zeile: FN
%           -4. Zeile: TN
%      -r_kamera: Matrix mit den Dimensionen 2,1:
%       Partikel die sich zum Zeitpunkt k*T auf dem Fließband befinden
%       aufgeteilt in Gutpartikel (1. Zeile) und Schlechtpartikel (2.Zeile)
%       (ist noch nicht aufgenommen, lässt sich aber eventuell hinzufügen)
%      -n_n: Steuerhorizont
%      -k_OV: Anzahl Zeitschritte, die ein Partikel benötigt, um die
%       Distanz zwischen Ausschleuseeinheit und Fließband zurückzulegen
%      -k_SO: Anzahl Zeitschritte, die ein Partikel benötigt, um die
%       Distanz zwischen Ausschleuseeinheit und Fließband zurückzulegen
%      -lb: lower bounds des Optimierungsvektors
%      -ub: upper bounds des Optimierungsvektors
%      -n_x: Anzahl Zustände + Regelgrößen (8)
%      -c_1, c_2: Gewichtungsfaktoren des Gütemaßes
%      -alpha, beta: W'keiten der Detektierung (siehe PDF)

%% Achtung
% -Teilweise gelten Bedingungen für n_n (müssen noch hinzugefügt werden)
% -Die Zustände und Stellgrößen starten zu unterschiedlichen Zeitpunkten
%  aufgrund der vielen Totzeiten

%% Optionen
options = optimoptions('fmincon', 'OptimalityTolerance', 1e-3,'Algorithm', 'sqp', ...
    'StepTolerance', 9.9e-5, 'MaxFunctionEvaluations', 1e6, 'MaxIterations', 1e6, 'ConstraintTolerance', 1e-2);
%% Parameter
% Prädiktionshorizont:
n_p = length(r_s);
n_n = int16(n_n);
if n_p < n_n
    r_s = [r_s, r_s(:,n_p).*ones(2,n_n-n_p)];
end
k_OK = int16(k_OK);


%% Nebenbedingungen
% lower bounds
lb = zeros(1,n_x*n_n)';

% upper bounds
ub_u = ones(1,(2*n_n));
ub = [ub_u Inf*ones(1, (n_x-2)*n_n)]';
% linear equality constraints
% Die if Struktur ist noetig, da bei groesseren Praediktionshorizonten
% (n_n) zusaetzliche nichtlineare Nebenbedingungen benoetigt werden, da die
% Zustaende nicht nur von bereits vergangenen Zeitpunkten und den
% Steuergroessen abhaengig sind
if n_n > k_OK
    beq = [r_s(1,1:k_OK)';r_s(2,1:k_OK)'];
    %           -u_P*y_TP                    -u_N*y_FN           x_P  
    Aeq_P = [-1*diag(y(1,1:k_OK)), zeros(k_OK,n_n-k_OK), -1*diag(y(3,1:k_OK)) zeros(k_OK,n_n-k_OK) eye(k_OK) zeros(k_OK,2*n_n-k_OK)];
    %           -u_P*y_FP                    -u_N*y_TN                    x_N   
    Aeq_N = [-1*diag(y(2,1:k_OK)), zeros(k_OK,n_n-k_OK), -1*diag(y(4,1:k_OK)), zeros(k_OK,2*n_n-k_OK),eye(k_OK), zeros(k_OK,n_n-k_OK)];
else
    beq = [r_s(1,1:n_n)';r_s(2,1:n_n)'];
    %           -u_P*y_TP                    -u_N*y_FN           x_P  
    Aeq_P = [-1*diag(y(1,1:n_n)) -1*diag(y(3,1:n_n)) eye(n_n) zeros(n_n)];
    %           -u_P*y_FP                    -u_N*y_TN                    x_N   
    Aeq_N = [-1*diag(y(2,1:n_n)), -1*diag(y(4,1:n_n)),zeros(n_n),eye(n_n)];
end
Aeq = [Aeq_P; Aeq_N];

% sparse Matrix ist zeitsparend
% Aeq_sparse = sparse(Aeq);
% beq_sparse = sparse(beq);
% Nichtlineare Nebenbedingungen
if n_n > k_OK
    [x_opt,~,exitflag,~] = fmincon(@(x)guetemass(x,n_n,c,alpha,beta, opt),x0,[],[],Aeq,beq,lb,ub,@(x)nonlincon(x,r_s, k_OK, n_n,alpha,beta),options);
else
    [x_opt,~,exitflag,~] = fmincon(@(x)guetemass(x,n_n,c,alpha,beta, opt),x0,[],[],Aeq,beq,lb,ub,[],options);
end
u_p = x_opt(1);
u_n = x_opt(n_n+1);
end

== matlab function library_schuettgut/Optischer Sortierer/Berechnung der stochastischen Matrix für die Sortiererwahrscheinlichkeiten/anteil_TN ==
  data: c_N input; TN_Anteil output
function TN_Anteil = anteil_TN(c_N)
%#codegen

%    This function was generated by the Symbolic Math Toolbox version 8.5.
%    23-Nov-2020 21:38:40

t2 = c_N.^2;
t3 = c_N.*1.216152772820919e-1;
t5 = c_N.*1.718305977216851e-4;
t4 = exp(t3);
t6 = -t5;
t7 = exp(t6);
TN_Anteil = ((c_N.*3.906219045425992e+17-t2.*4.590953499729531e+15+1.319829183465711e+20).*(c_N.*7.378697629483821e+19-t4.*9.913820620264122e+16+t7.*7.377089983858165e+21-7.378697629483821e+21).*(-2.710505431213761e-20))./(c_N.*(c_N.*-7.812438090851985e+17+t2.*9.181906999459062e+15+t4.*3.965528248105649e+15-t7.*2.950835993543266e+20+3.118206848621062e+19));

== matlab function library_schuettgut/Optischer Sortierer/Berechnung der stochastischen Matrix für die Sortiererwahrscheinlichkeiten/anteil_TP ==
  data: c_N input; TP_Anteil output
function TP_Anteil = anteil_TP(c_N)
%#codegen

%    This function was generated by the Symbolic Math Toolbox version 8.5.
%    23-Nov-2020 21:35:04

t2 = c_N.^2;
t3 = c_N.*1.216152772820919e-1;
t5 = c_N.*1.718305977216851e-4;
t4 = exp(t3);
t6 = -t5;
t7 = exp(t6);
t8 = t4.*3.965528248105649e+15;
t9 = t7.*2.950835993543266e+20;
t10 = -t9;
TP_Anteil = ((t8+t10).*(c_N.*2.712794053385412e+19+t2.*1.147738374932383e+17-3.299572958664278e+21).*1.965116437629977e-18)./((c_N.*(1.45e+2./2.0)-7.25e+3).*(c_N.*-7.812438090851985e+17+t2.*9.181906999459062e+15+t8+t10+3.118206848621062e+19));

== matlab function library_schuettgut/decomposition_gTV ==
  data: x1 input; g output; x2 input
function g = decomposition_gTV(x1,x2)
%#codegen

%    This function was generated by the Symbolic Math Toolbox version 8.5.
%    26-Jan-2021 10:32:40

t2 = conj(x1);
t3 = conj(x2);
g = [t2.*(-6.586048041173689e-2)+t2.^2.*7.024962657286325e-5;t3.*(-1.448698496758973e-1)-t3.^2.*4.647981435157282e-3];

== matlab function library_schuettgut/Optischer SortiererV2/Berechnung der stochastischen Matrix für die Sortiererwahrscheinlichkeiten/epsilon_test ==
  data: xp input; y output; xn input
function y = fcn(xp,xn)
p1 =   -0.003787;
p2 =     0.05479;
p3 =      0.6837;
p4 = -0.007;
y = p1*(xp+xn)^2 + p2*(xp+xn) + p3 +p4*xn;
end

== matlab function library_schuettgut/Optischer SortiererV2/Berechnung der stochastischen Matrix für die Sortiererwahrscheinlichkeiten/zeta_test ==
  data: xp input; y output; xn input
function y = fcn(xp,xn)
p1 =   -0.003787;
p2 =     0.05479;
p3 =      0.5837;
p4 = 0.007;
y = p1*(xp+xn)^2 + p2*(xp+xn) + p3 +p4*xn;
end
